simulink model "Nonadaptive_Open_loop_rotor_flux_observer"  (R2021a)
settings: Solver=FixedStepDiscrete  StartTime=0.0  StopTime=10.0  FixedStep=1E-05  RelTol=1e-3
undefined symbols (not defined in the file): DiscIntNeverNeededParam
settings Model: Creator=Mehra  LastModifiedBy=Mehra

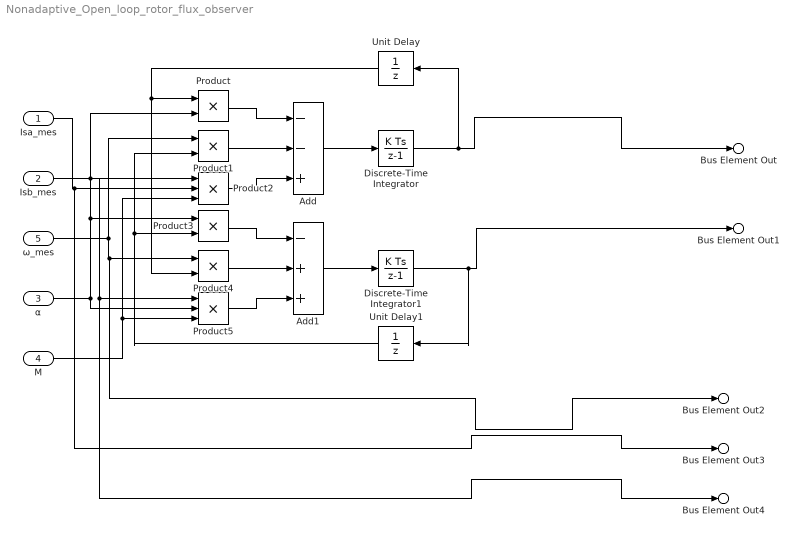
== system Nonadaptive_Open_loop_rotor_flux_observer ==
  Isa_mes : Inport
  Isb_mes : Inport  Port=2
  α : Inport  Port=3
  M : Inport  Port=4
  ω_mes : Inport  Port=5
  Add : Sum  Inputs=--+
  Add1 : Sum  Inputs=-++
  Discrete-Time Integrator : DiscreteIntegrator  SampleTime=-1  ICPrevOutput=DiscIntNeverNeededParam  ICPrevScaledInput=DiscIntNeverNeededParam
  Discrete-Time Integrator1 : DiscreteIntegrator  SampleTime=-1  ICPrevOutput=DiscIntNeverNeededParam  ICPrevScaledInput=DiscIntNeverNeededParam
  Product{,1,3..4} (4 alike) : Product
  Product2 : Product  Inputs=3
  Product5 : Product  Inputs=3
  Unit Delay : UnitDelay  SampleTime=-1  HasFrameUpgradeWarning=on
  Unit Delay1 : UnitDelay  SampleTime=-1  HasFrameUpgradeWarning=on
  Bus Element Out : Outport  PortName=mes  Element=Ψra
  Bus Element Out1 : Outport  PortName=mes  Element=Ψrb
  Bus Element Out2 : Outport  PortName=mes  Element=ω
  Bus Element Out3 : Outport  PortName=mes  Element=Isa
  Bus Element Out4 : Outport  PortName=mes  Element=Isb
  wires:
  Product/1 -> Add/1
  Product1/1 -> Add/2
  Product2/1 -> Add/3
  Product3/1 -> Add1/1
  Product4/1 -> Add1/2
  Product5/1 -> Add1/3
  Add/1 -> Discrete-Time Integrator/1
  Discrete-Time Integrator/1 -> Unit Delay/1, Bus Element Out/1
  α/1 -> Product5/2, Product2/1, Product/2, Product3/1
  ω_mes/1 -> Bus Element Out2/1, Product4/1, Product1/1
  Add1/1 -> Discrete-Time Integrator1/1
  Discrete-Time Integrator1/1 -> Unit Delay1/1, Bus Element Out1/1
  Isa_mes/1 -> Bus Element Out3/1, Product2/2
  M/1 -> Product5/3, Product2/3
  Isb_mes/1 -> Product5/1, Bus Element Out4/1
  Unit Delay/1 -> Product/1, Product4/2
  Unit Delay1/1 -> Product1/2, Product3/2
